simulink model "s1_cserbatoio"  (Simulink 10.0)
settings: Solver=ode45  StartTime=0.0  StopTime=24  RelTol=1e-3  AbsTol=1e-6
settings Model: Creator=AR  LastModifiedBy=AR  ExtModeTrigMode=oneshot  ExtModeArmWhenConnect=off
settings DataIOCC: SignalLoggingSaveFormat=ModelDataLogs  SignalLoggingName=sigsOut
settings OptimizationCC: BooleanDataType=off  LifeSpan=auto
settings DebuggingCC: SaveWithParameterizedLinksMsg=none  SignalResolutionControl=TryResolveAllWithWarning  MultiTaskDSMMsg=warning  MultiTaskCondExecSysMsg=none  SFUnexpectedBacktrackingDiag=error  SFNoUnconditionalDefaultTransitionDiag=error  SFExecutionAtInitializationDiag=warning  ArithmeticOperatorsInVariantConditions=error
settings HardwareCC: TargetUnknown=on
settings SFSimCC: SimUseLocalCustomCode=on  CustomCodeUndefinedFunction=FilterOut
settings RTWCC: RTWUseLocalCustomCode=on
settings CodeAppCC: StateflowObjectComments=off
settings GRTTargetCC: TargetLangStandard=C99 (ISO)

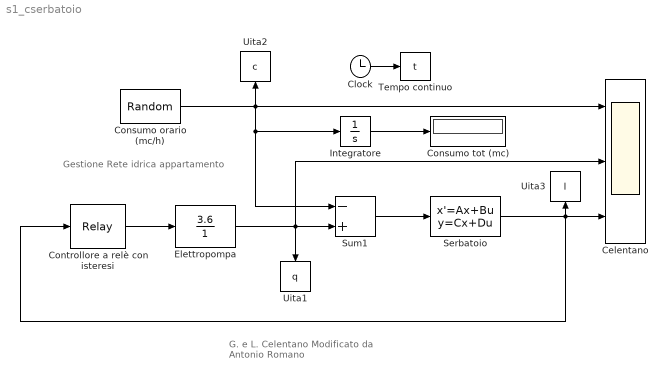
== system s1_cserbatoio ==
  note: Gestione Rete idrica appartamento
  note: G. e L. Celentano
      | Modificato da Antonio Romano
  Celentano : Scope  NumInputPorts=3
  Clock : Clock
  Consumo orario (mc/h) : RandomNumber  Mean=0.03667  Variance=0.3^2  SampleTime=1
  Consumo tot (mc) : Display
  Controllore a relè con isteresi : Relay  OnSwitchValue=10  OffSwitchValue=7  OnOutputValue=0  OffOutputValue=1
  Elettropompa : TransferFcn  Numerator=3.6  Denominator=[1]
  Integratore : Integrator
  Serbatoio : StateSpace  A=0  B=1/1.1289  D=0  InitialCondition=6.5
  Sum1 : Sum  Inputs=-+  SaturateOnIntegerOverflow=on  InputSameDT=on  OutDataTypeStr=Inherit: Same as first input
  Tempo continuo : ToWorkspace  VariableName=t  SampleTime=-1
  Uita1 : ToWorkspace  VariableName=q  SampleTime=-1
  Uita2 : ToWorkspace  VariableName=c  SampleTime=-1
  Uita3 : ToWorkspace  VariableName=l  SampleTime=-1
  wires:
  Consumo orario (mc/h)/1 -> Celentano/1, Uita2/1, Integratore/1, Sum1/1
  Integratore/1 -> Consumo tot (mc)/1
  Serbatoio/1 -> Controllore a relè con isteresi/1, Celentano/3, Uita3/1
  Clock/1 -> Tempo continuo/1
  Sum1/1 -> Serbatoio/1
  Controllore a relè con isteresi/1 -> Elettropompa/1
  Elettropompa/1 -> Sum1/2, Celentano/2, Uita1/1
